simulink model "FDCAN_GATEWAY"  (R2024b)
settings: Solver=FixedStepAuto  StartTime=0.0  StopTime=10.0  RelTol=1e-3  EnableMultiTasking=on
undefined symbols (not defined in the file): CAN, FD
libraries: stmutilitieslib x11, stm32blockslib x9, canmsglib x3, stm32f4xxblockslib x1, dlcombinationlib x1
settings Model: STM32="{\"FDCANWrite\":[{\"ID\":\"FDCAN_GATEWAY:3\"},{\"ID\":\"FDCAN_GATEWAY:18\"},{\"ID\":\"FDCAN_GATEWAY:25\"},{\"ID\":\"FDCAN_GATEWAY:70\"},{\"ID\":\"FDCAN_GATEWAY:71\"},{\"ID\":\"FDCAN_GATEWAY:72\"},{\"ID\":\"FDCAN_GATEWAY:74\"}],\"FDCANRead\":[{\"ID\":\"FDCAN_GATEWAY:7\"},{\"ID\":\"FDCAN_GATEWAY:23\"}],\"DigitalPortWrite\":{\"ID\":\"FDCAN_GATEWAY:27\"}}"  Creator=aferreira  LastModifiedBy=aferreira
settings SolverCC: PositivePriorityOrder=on
settings OptimizationCC: EnhancedBackFolding=on  PassReuseOutputArgsAs=Individual arguments  ZeroExternalMemoryAtStartup=off  ZeroInternalMemoryAtStartup=off  MaxStackSize=64  OptimizeBlockOrder=speed  DifferentSizesBufferReuse=on  OptimizationCustomize=off  EfficientTunableParamExpr=on
settings DebuggingCC: ParameterTunabilityLossMsg=error  UnderSpecifiedDimensionMsg=warning
settings HardwareCC: ProdBitPerPointer=32  ProdBitPerSizeT=32  ProdBitPerPtrDiffT=32  ProdLargestAtomicInteger=Long  ProdLargestAtomicFloat=Double  ProdWordSize=32  ProdLongLongMode=on  ProdHWDeviceType=ARM Compatible->ARM Cortex-M
settings SFSimCC: MATLABDynamicMemAlloc=off
settings RTWCC: Description=Embedded Coder  SystemTargetFile=ert.tlc  HardwareBoard=STM32H7xx Based (Single-core)  TLCOptions="-aInlineSetEventsForThisBaseRateFcn=TLC_FALSE -aSuppressMultiTaskScheduler=TLC_FALSE  -aRateBasedStepFcn=0"  TemplateMakefile=ert_default_tmf  Toolchain=GNU Tools for ARM Embedded Processors
settings CodeAppCC: ForceParamTrailComments=on  IgnoreCustomStorageClasses=off  OperatorAnnotations=on  SimulinkDataObjDesc=on  SFDataObjDesc=on  InsertBlockDesc=on
settings ERTTargetCC: TargetLangStandard=C99 (ISO)  CodeReplacementLibrary=ARM Cortex-M  ExtModeTransport=3  ExtModeStaticAlloc=on  ExtModeStaticAllocSize=2048  ExtModeMexFile=ext_xcp  ExtModeIntrfLevel=Level2 - Open  InlinedParameterPlacement=Hierarchical  DynamicArrayContainerType=coder::array

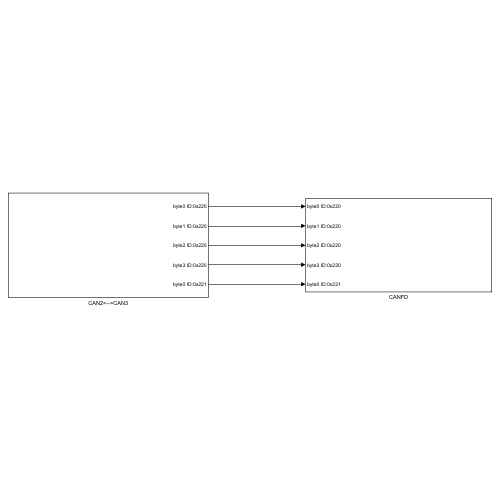
[thumbnail: Simulink's stored preview of the top-level diagram]
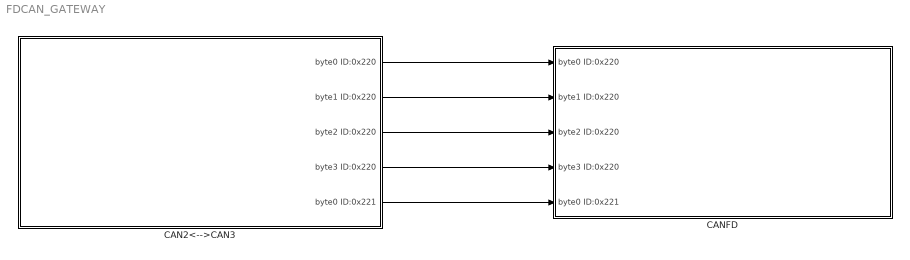
== system FDCAN_GATEWAY ==
  CAN2<-->CAN3 : Subsystem
  CANFD : Subsystem
  wires:
  CAN2<-->CAN3/1(byte0 ID:0x220) -> CANFD/1(byte0 ID:0x220)
  CAN2<-->CAN3/2(byte1 ID:0x220) -> CANFD/2(byte1 ID:0x220)
  CAN2<-->CAN3/3(byte2 ID:0x220) -> CANFD/3(byte2 ID:0x220)
  CAN2<-->CAN3/4(byte3 ID:0x220) -> CANFD/4(byte3 ID:0x220)
  CAN2<-->CAN3/5(byte0 ID:0x221) -> CANFD/5(byte0 ID:0x221)

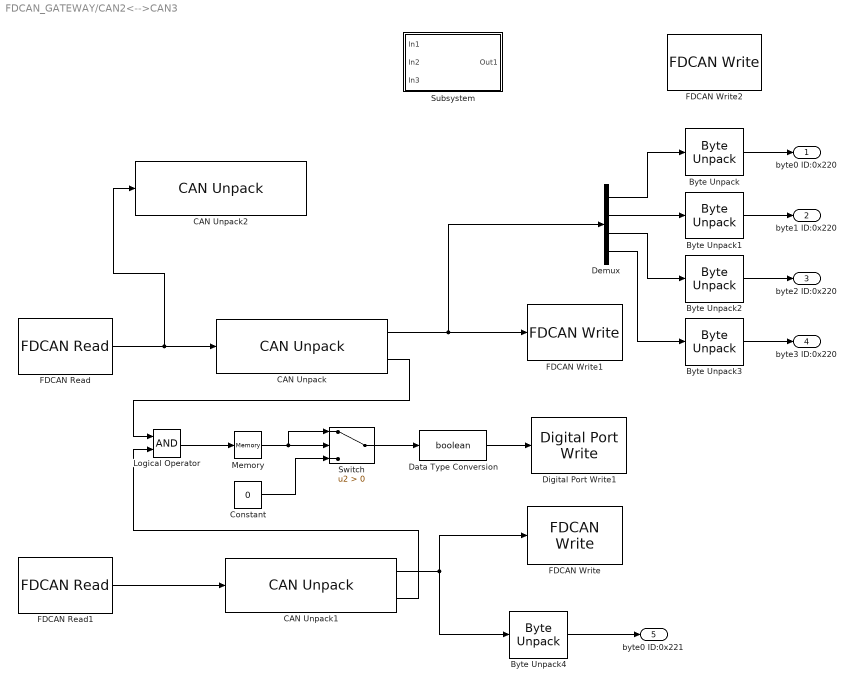
== system FDCAN_GATEWAY/CAN2<-->CAN3 ==
  Byte Unpack{,1..4} (5 alike) : stmutilitieslib/Byte Unpack  dimensions={[1]}  datatypes={'uint8'}  byteAlign=1  blockPlatform=stm32f4discovery
  CAN Unpack : canmsglib/CAN Unpack  MsgList=(none)  MsgName=CAN Msg  MsgIDType=Standard (11-bit identifier)  MsgIdentifier=0x220  MsgLength=4  SignalInfo={}  IDPort=off  TimestampPort=off  ErrorPort=off  RemotePort=off  LengthPort=off  StatusPort=on  ApplyMinMax=off
      settings: LibrarySourceBlock=stmutilitieslib/CAN Unpack  DataFormat=raw data
  CAN Unpack1 : canmsglib/CAN Unpack  MsgList=(none)  MsgName=CAN Msg  MsgIDType=Standard (11-bit identifier)  MsgIdentifier=0x221  MsgLength=1  SignalInfo={}  IDPort=off  TimestampPort=off  ErrorPort=off  RemotePort=off  LengthPort=off  StatusPort=on  ApplyMinMax=off
      settings: LibrarySourceBlock=stmutilitieslib/CAN Unpack  DataFormat=raw data
  CAN Unpack2 : canmsglib/CAN Unpack  MsgList=(none)  MsgName=CAN Msg  MsgIDType=Standard (11-bit identifier)  MsgIdentifier=0x226  MsgLength=6  SignalInfo={}  IDPort=off  TimestampPort=off  ErrorPort=off  RemotePort=off  LengthPort=off  StatusPort=off  ApplyMinMax=off
      settings: LibrarySourceBlock=stmutilitieslib/CAN Unpack  DataFormat=raw data
  Constant : Constant  Value=0
  Data Type Conversion : DataTypeConversion  OutDataTypeStr=boolean  SaturateOnIntegerOverflow=off  RndMeth=Floor
  Demux : Demux
  Digital Port Write1 : stm32f4xxblockslib/Digital Port Write  PortName=GPIOD  PinNumber=[3]  ReadOperation=off  IOAsArray=on  EnableSimPort=off  hoistedMaskSrc=ECSoC/ECSimCodegen/Digital Port Write
      settings: LibrarySourceBlock=stm32h7xxblockslib/Digital Port Write
  FDCAN Read : stm32blockslib/FDCAN Read  FDCANModule=FDCAN2  BlockMode=Receive  OperationReadMode=Data  OperationWriteMode=Data  ReadSource=FIFO 0  BufferNumber=0  OutputTypeReadMode=Packed  DataFormatWriteMode=Raw data  CANFrameType=CAN-FD  IdentifierTypeVia=Dialog  IdentifierType=Standard (11-bit identifier)  IdentifierVia=Inport  Identifier=100  DataLengthVia=Inport  DataLength=64  OutputIdType=off  IsBitRateSwitchingEnabled=off  TransmitRemoteFrame=off  OutputFrameType=off  OutputBRS=off  OutputRemoteFrame=off  OutputTxFifoLevel=off  OutputRxFifoLevel=off  OutputStatus=off  Timeout=0.001  SampleTime=0.001
      settings: LibrarySourceBlock=stm32g4xxblockslib/FDCAN Read
  FDCAN Read1 : stm32blockslib/FDCAN Read  FDCANModule=FDCAN3  BlockMode=Receive  OperationReadMode=Data  OperationWriteMode=Data  ReadSource=FIFO 0  BufferNumber=0  OutputTypeReadMode=Packed  DataFormatWriteMode=Raw data  CANFrameType=CAN-FD  IdentifierTypeVia=Dialog  IdentifierType=Standard (11-bit identifier)  IdentifierVia=Inport  Identifier=100  DataLengthVia=Inport  DataLength=64  OutputIdType=off  IsBitRateSwitchingEnabled=off  TransmitRemoteFrame=off  OutputFrameType=off  OutputBRS=off  OutputRemoteFrame=off  OutputTxFifoLevel=off  OutputRxFifoLevel=off  OutputStatus=off  Timeout=0.001  SampleTime=0.001
      settings: LibrarySourceBlock=stm32g4xxblockslib/FDCAN Read
  FDCAN Write : stm32blockslib/FDCAN Write  FDCANModule=FDCAN2  BlockMode=Transmit  OperationReadMode=Data  OperationWriteMode=Data  ReadSource=FIFO 0  BufferNumber=0  OutputTypeReadMode=Unpacked  DataFormatWriteMode=Raw data  CANFrameType=CAN  IdentifierTypeVia=Dialog  IdentifierType=Standard (11-bit identifier)  IdentifierVia=Dialog  Identifier=0x221  DataLengthVia=Dialog  DataLength=1  OutputIdType=off  IsBitRateSwitchingEnabled=off  TransmitRemoteFrame=off  OutputFrameType=off  OutputBRS=off  OutputRemoteFrame=off  OutputTxFifoLevel=off  OutputRxFifoLevel=off  OutputStatus=off  Timeout=0.001  SampleTime=-1
      settings: LibrarySourceBlock=stm32g4xxblockslib/FDCAN Write
  FDCAN Write1 : stm32blockslib/FDCAN Write  FDCANModule=FDCAN3  BlockMode=Transmit  OperationReadMode=Data  OperationWriteMode=Data  ReadSource=FIFO 0  BufferNumber=0  OutputTypeReadMode=Unpacked  DataFormatWriteMode=Raw data  CANFrameType=CAN  IdentifierTypeVia=Dialog  IdentifierType=Standard (11-bit identifier)  IdentifierVia=Dialog  Identifier=0x220  DataLengthVia=Dialog  DataLength=4  OutputIdType=off  IsBitRateSwitchingEnabled=off  TransmitRemoteFrame=off  OutputFrameType=off  OutputBRS=off  OutputRemoteFrame=off  OutputTxFifoLevel=off  OutputRxFifoLevel=off  OutputStatus=off  Timeout=0.001  SampleTime=-1
      settings: LibrarySourceBlock=stm32g4xxblockslib/FDCAN Write
  FDCAN Write2 : stm32blockslib/FDCAN Write  FDCANModule=FDCAN3  BlockMode=Transmit  OperationReadMode=Data  OperationWriteMode=Data  ReadSource=FIFO 0  BufferNumber=0  OutputTypeReadMode=Unpacked  DataFormatWriteMode=Raw data  CANFrameType=CAN  IdentifierTypeVia=Dialog  IdentifierType=Standard (11-bit identifier)  IdentifierVia=Dialog  Identifier=0x226  DataLengthVia=Dialog  DataLength=3  OutputIdType=off  IsBitRateSwitchingEnabled=off  TransmitRemoteFrame=off  OutputFrameType=off  OutputBRS=off  OutputRemoteFrame=off  OutputTxFifoLevel=off  OutputRxFifoLevel=off  OutputStatus=off  Timeout=0.001  SampleTime=-1
      settings: LibrarySourceBlock=stm32g4xxblockslib/FDCAN Write
  Logical Operator : Logic  AllPortsSameDT=off  OutDataTypeStr=boolean
  Memory : Memory
  Subsystem : Subsystem
  Switch : Switch  Criteria=u2 > Threshold  SaturateOnIntegerOverflow=off  InputSameDT=off
  byte0 ID:0x220 : Outport  OutDataTypeStr=uint8
  byte1 ID:0x220 : Outport  Port=2  OutDataTypeStr=uint8
  byte2 ID:0x220 : Outport  Port=3  OutDataTypeStr=uint8
  byte3 ID:0x220 : Outport  Port=4  OutDataTypeStr=uint8
  byte0 ID:0x221 : Outport  Port=5
  wires:
  FDCAN Read/1 -> CAN Unpack2/1, CAN Unpack/1
  CAN Unpack/1 -> Demux/1, FDCAN Write1/1
  FDCAN Read1/1 -> CAN Unpack1/1
  CAN Unpack1/1 -> FDCAN Write/1, Byte Unpack4/1
  Data Type Conversion/1 -> Digital Port Write1/1
  Constant/1 -> Switch/3
  Switch/1 -> Data Type Conversion/1
  CAN Unpack/2 -> Logical Operator/1
  CAN Unpack1/2 -> Logical Operator/2
  Logical Operator/1 -> Memory/1
  Memory/1 -> Switch/1, Switch/2
  Demux/1 -> Byte Unpack/1
  Demux/2 -> Byte Unpack1/1
  Demux/3 -> Byte Unpack2/1
  Demux/4 -> Byte Unpack3/1
  Byte Unpack/1 -> byte0 ID:0x220/1
  Byte Unpack1/1 -> byte1 ID:0x220/1
  Byte Unpack2/1 -> byte2 ID:0x220/1
  Byte Unpack3/1 -> byte3 ID:0x220/1
  Byte Unpack4/1 -> byte0 ID:0x221/1

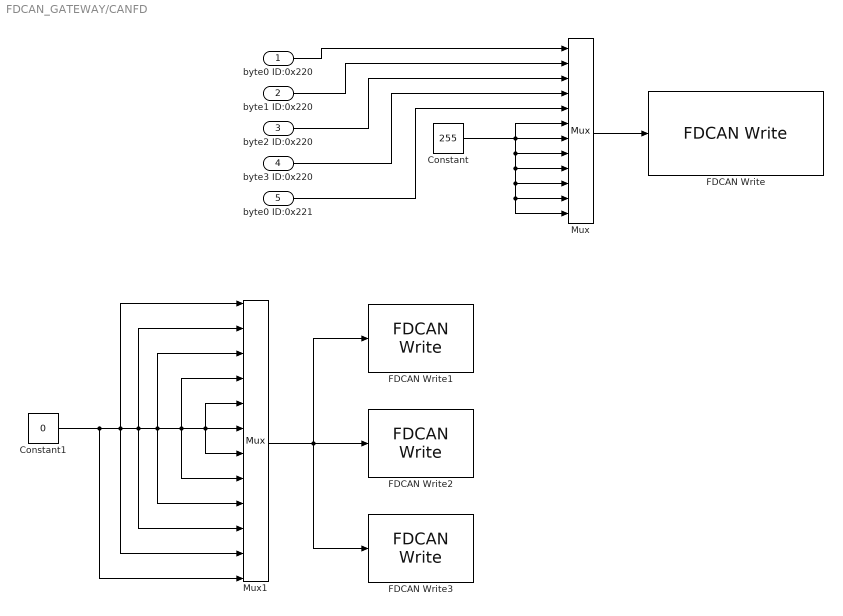
== system FDCAN_GATEWAY/CANFD ==
  byte0 ID:0x220 : Inport  OutDataTypeStr=uint8
  byte1 ID:0x220 : Inport  Port=2  OutDataTypeStr=uint8
  byte2 ID:0x220 : Inport  Port=3  OutDataTypeStr=uint8
  byte3 ID:0x220 : Inport  Port=4  OutDataTypeStr=uint8
  byte0 ID:0x221 : Inport  Port=5  OutDataTypeStr=uint8
  Constant : Constant  Value=255  OutDataTypeStr=uint8
  Constant1 : Constant  Value=0  OutDataTypeStr=uint8
  FDCAN Write : stm32blockslib/FDCAN Write  FDCANModule=FDCAN1  BlockMode=Transmit  OperationReadMode=Data  OperationWriteMode=Data  ReadSource=FIFO 0  BufferNumber=0  OutputTypeReadMode=Unpacked  DataFormatWriteMode=Raw data  CANFrameType=CAN-FD  IdentifierTypeVia=Dialog  IdentifierType=Standard (11-bit identifier)  IdentifierVia=Dialog  Identifier=0x223  DataLengthVia=Dialog  DataLength=12  OutputIdType=off  IsBitRateSwitchingEnabled=off  TransmitRemoteFrame=off  OutputFrameType=off  OutputBRS=off  OutputRemoteFrame=off  OutputTxFifoLevel=off  OutputRxFifoLevel=off  OutputStatus=off  Timeout=0.001  SampleTime=-1
      settings: LibrarySourceBlock=stm32g4xxblockslib/FDCAN Write
  FDCAN Write1 : stm32blockslib/FDCAN Write  FDCANModule=FDCAN1  BlockMode=Transmit  OperationReadMode=Data  OperationWriteMode=Data  ReadSource=FIFO 0  BufferNumber=0  OutputTypeReadMode=Unpacked  DataFormatWriteMode=Raw data  CANFrameType=CAN-FD  IdentifierTypeVia=Dialog  IdentifierType=Standard (11-bit identifier)  IdentifierVia=Dialog  Identifier=0x224  DataLengthVia=Dialog  DataLength=12  OutputIdType=off  IsBitRateSwitchingEnabled=off  TransmitRemoteFrame=off  OutputFrameType=off  OutputBRS=off  OutputRemoteFrame=off  OutputTxFifoLevel=off  OutputRxFifoLevel=off  OutputStatus=off  Timeout=0.001  SampleTime=-1
      settings: LibrarySourceBlock=stm32h7xxblockslib/FDCAN Write
  FDCAN Write2 : stm32blockslib/FDCAN Write  FDCANModule=FDCAN1  BlockMode=Transmit  OperationReadMode=Data  OperationWriteMode=Data  ReadSource=FIFO 0  BufferNumber=0  OutputTypeReadMode=Unpacked  DataFormatWriteMode=Raw data  CANFrameType=CAN-FD  IdentifierTypeVia=Dialog  IdentifierType=Standard (11-bit identifier)  IdentifierVia=Dialog  Identifier=0x225  DataLengthVia=Dialog  DataLength=12  OutputIdType=off  IsBitRateSwitchingEnabled=off  TransmitRemoteFrame=off  OutputFrameType=off  OutputBRS=off  OutputRemoteFrame=off  OutputTxFifoLevel=off  OutputRxFifoLevel=off  OutputStatus=off  Timeout=0.001  SampleTime=-1
      settings: LibrarySourceBlock=stm32h7xxblockslib/FDCAN Write
  FDCAN Write3 : stm32blockslib/FDCAN Write  FDCANModule=FDCAN1  BlockMode=Transmit  OperationReadMode=Data  OperationWriteMode=Data  ReadSource=FIFO 0  BufferNumber=0  OutputTypeReadMode=Unpacked  DataFormatWriteMode=Raw data  CANFrameType=CAN-FD  IdentifierTypeVia=Dialog  IdentifierType=Standard (11-bit identifier)  IdentifierVia=Dialog  Identifier=0x226  DataLengthVia=Dialog  DataLength=12  OutputIdType=off  IsBitRateSwitchingEnabled=off  TransmitRemoteFrame=off  OutputFrameType=off  OutputBRS=off  OutputRemoteFrame=off  OutputTxFifoLevel=off  OutputRxFifoLevel=off  OutputStatus=off  Timeout=0.001  SampleTime=-1
      settings: LibrarySourceBlock=stm32h7xxblockslib/FDCAN Write
  Mux : Mux  Inputs=12
  Mux1 : Mux  Inputs=12
  wires:
  Mux/1 -> FDCAN Write/1
  byte0 ID:0x220/1 -> Mux/1
  byte1 ID:0x220/1 -> Mux/2
  byte2 ID:0x220/1 -> Mux/3
  byte3 ID:0x220/1 -> Mux/4
  byte0 ID:0x221/1 -> Mux/5
  Constant/1 -> Mux/12, Mux/11, Mux/10, Mux/9, Mux/8, Mux/7, Mux/6
  Constant1/1 -> Mux1/12, Mux1/1, Mux1/11, Mux1/2, Mux1/10, Mux1/3, Mux1/9, Mux1/4, Mux1/8, Mux1/7, Mux1/5, Mux1/6
  Mux1/1 -> FDCAN Write3/1, FDCAN Write2/1, FDCAN Write1/1

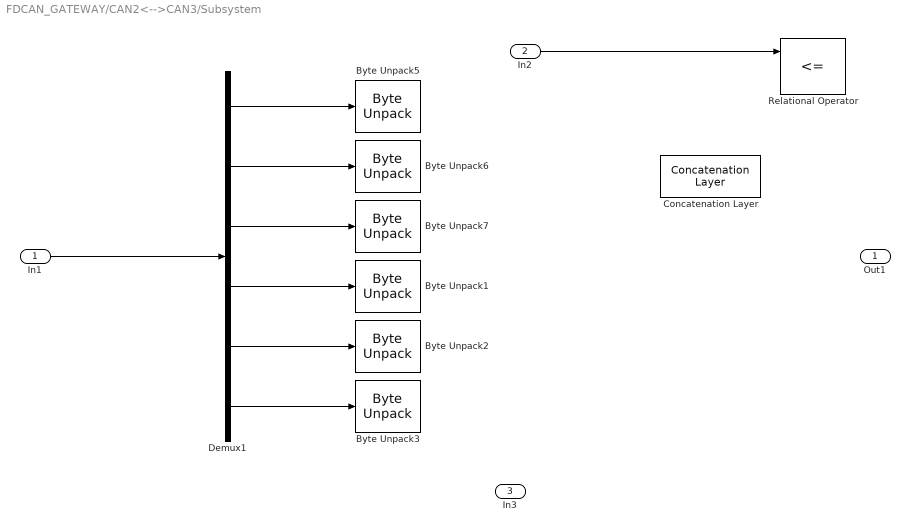
== system FDCAN_GATEWAY/CAN2<-->CAN3/Subsystem ==
  In1 : Inport
  In2 : Inport  Port=2
  In3 : Inport  Port=3
  Byte Unpack{1..3,5..7} (6 alike) : stmutilitieslib/Byte Unpack  dimensions={[1]}  datatypes={'uint8'}  byteAlign=1  blockPlatform=stm32f4discovery
  Concatenation Layer : dlcombinationlib/Concatenation Layer  Layer=layer  SampleTime=-1
      settings: DataFormat=SSC
  Demux1 : Demux  Outputs=6
  Relational Operator : RelationalOperator  Operator=<=  OutDataTypeStr=boolean  RndMeth=Simplest  InputSameDT=off
  Out1 : Outport
  wires:
  In1/1 -> Demux1/1
  Demux1/1 -> Byte Unpack5/1
  Demux1/2 -> Byte Unpack6/1
  Demux1/3 -> Byte Unpack7/1
  Demux1/4 -> Byte Unpack1/1
  Demux1/5 -> Byte Unpack2/1
  Demux1/6 -> Byte Unpack3/1
  In2/1 -> Relational Operator/1
